simulink library "carnotUIBK"  (R2024b)
settings: Solver=VariableStepAuto  StartTime=0.0  StopTime=10.0  RelTol=1e-3  EnableMultiTasking=on
values from neighbouring files (symbols this model uses):
  area = area + room(kk).area    [THERMALZONE.m]
  boundary = BOUNDARY()    [BUILDING.m]
  building = obj    [BUILDING.m]
  C = zeros(1,length(d)+1)    [CONSTRUCTION.m]
  cp = str2num(value)    [CONSTRUCTION.m]
  pos = find(d_layer>0)    [CONSTRUCTION.m]
  rho = str2num(value)    [CONSTRUCTION.m]
  type = 1    [CONSTRUCTION.m]
  zone = obj.zone(ind)    [THERMALZONE.m]
undefined symbols (not defined in the file or in its folder): A, amb_factor, B, const, control, Dd, get_building, height, p, Qdot_C, Qdot_H, Qdot_I_electricity, Qdot_I_light, Qdot_I_person, Qdot_S, Qdot_T_ground, Qdot_T_neighbour, Qdot_T_opaque, Qdot_T_window, Qdot_V_infiltration, Qdot_V_mech, Qdot_V_window, r_frame, solar_ratio, solar_ratio1, solar_ratio2, Tc, Tr, Ts, Uvalue, view_factor, wall, wallsurface, window, window_height, window_heigth, window_width, windowsurface, x_CO2, x_H2O, x_VOC, z
libraries: carnot x105, $bdroot x22, simulink x18, simulink_extras x14
(part 8 of 13)

== system carnotUIBK/window/window_CARNOT/alfa_window_in ==
  note: (W/m^2)
  note: CONVENTION:
      | Qdot > 0 and qdots < 0, if Ts > T (heat flows from wall surface to room node),
      | Qdot < 0 and qdots > 0, if Ts < T (heat flows from room node to wall surface).
  note: s: surface
      | c: convective
      | r: radiative
  note: WINDOW = FRAME + GLASS
  note: (W/m^2)
  note: Convective and radiative heat transfer at the INDOOR SURFACE OF A VERTICAL WINDOW
      | with 1-4 layers (each 3 ... 8 mm thick)
  note: (°C)
  Ts2 : Inport
  "[sun_t]" : Inport  Port=2
  "[AIV]" : Inport  Port=3
  Demux : Demux  Outputs=[1 1 1 6]
      settings: DisplayOption=none
  Demux1 : Demux  Outputs=[1 2]
      settings: DisplayOption=none
  Ground2 : Ground
  Ground3 : Ground
  Ground4 : Ground
  Irradiation into room : Subsystem
  Mux : Mux  Inputs=2
  Mux4 : Mux  Inputs=[2 1 2 2 12]
  Product5 : Product  InputSameDT=on  SaturateOnIntegerOverflow=on  OutDataTypeStr=Inherit: Same as first input
  Sum : Sum  Inputs=-+  InputSameDT=on  SaturateOnIntegerOverflow=on  OutDataTypeStr=Inherit: Same as first input
  Sum1 : Sum  Inputs=+-  InputSameDT=on  SaturateOnIntegerOverflow=on  OutDataTypeStr=Inherit: Same as first input
  Sum2 : Sum  Inputs=--  InputSameDT=on  SaturateOnIntegerOverflow=on  OutDataTypeStr=Inherit: Same as first input
  Terminator : Terminator
  Terminator1 : Terminator
  emission_in : Gain  Gain=emission_in  SaturateOnIntegerOverflow=on  OutDataTypeStr=Inherit: Same as input  ParamDataTypeStr=Inherit: Same as input
  surface of window : Gain  Gain=wallsurface  SaturateOnIntegerOverflow=on  OutDataTypeStr=Inherit: Same as input  ParamDataTypeStr=Inherit: Same as input
  surface of window glass : Gain  Gain=(1-frame)*wallsurface  SaturateOnIntegerOverflow=on  OutDataTypeStr=Inherit: Same as input  ParamDataTypeStr=Inherit: Same as input
  transmission coefficient 1-2-3-4-layer(s) : Subsystem
  u_convection : Gain  Gain=2.5  SaturateOnIntegerOverflow=on  OutDataTypeStr=Inherit: Same as input  ParamDataTypeStr=Inherit: Same as input
  u_rad : Constant  Value=5.6
  u_rad1 : Constant  Value=zeros(numlayer,1)
  qdots2 : Outport  InitialOutput=0  VectorParamsAs1DForOutWhenUnconnected=off
  qdot_abs : Outport  Port=2  InitialOutput=0  VectorParamsAs1DForOutWhenUnconnected=off
  "[S]" : Outport  Port=3  InitialOutput=0  VectorParamsAs1DForOutWhenUnconnected=off
  wires:
  Sum2/1 -> qdots2/1
  Demux/4 -> Terminator1/1
  "[AIV]"/1 -> Demux/1
  Demux/1 -> Terminator/1
  Mux/1 -> surface of window/1
  emission_in/1 -> Product5/1
  Sum1/1 -> Product5/2  "dTr"
  u_rad/1 -> emission_in/1
  Ts2/1 -> Sum/2, Sum1/1  "Ts"
  Product5/1 -> Mux/2, Sum2/2  "qdotr"
  u_convection/1 -> Sum2/1, Mux/1  "qdotc"
  Irradiation into room/1(qdot_sol) -> surface of window glass/1  "qdot_sol (>= 0)"
  Demux1/1 -> transmission coefficient 1-2-3-4-layer(s)/1(teta)  "teta"
  "[sun_t]"/1 -> Demux1/1
  Demux/2 -> Sum/1  "Tc"
  u_rad1/1 -> qdot_abs/1
  Sum/1 -> u_convection/1  "dTc"
  Demux/3 -> Sum1/2  "Tr"
  Demux1/2 -> Irradiation into room/1("[I_t]")  "[I_t]"
  transmission coefficient 1-2-3-4-layer(s)/1("[tau]") -> Irradiation into room/2("[tau]")
  Mux4/1 -> "[S]"/1
  Ground3/1 -> Mux4/5
  Ground2/1 -> Mux4/4
  Ground4/1 -> Mux4/3
  surface of window/1 -> Mux4/1  "[Qdotc, Qdotr]"
  surface of window glass/1 -> Mux4/2  "Qdot_sol"

== system carnotUIBK/window/window_CARNOT/alfa_window_out ==
  note: WINDOW = FRAME + GLASS
  note: Convective and radiative heat transfer at the OUTDOOR SURFACE OF A VERTICAL WINDOW
  note: modified
      | weatherdata
  note: s: surface
      | c: convective
      | r: radiative
      | h: in height
      | t: tilted surface
  note: CONVENTION:
      | qdots < 0, if Ts > T, heat flows from window surface (resp. room node) to ambition,
      | qdots > 0, if Ts < T, heat flows from ambition to window surface (resp. room node).
  WDB : Inport
  g : Inport  Port=2
  Ts1 : Inport  Port=3
  Bus Selector : BusSelector  OutputSignals=Temperature_Ambient,Temperature_Sky_Radiation,Wind_Speed
  Bus Selector1 : BusSelector  OutputSignals=Incidence_Angle_sun,Solar_Radiation_direct_surface,Solar_Radiation_diffuse_surface
  Ground1 : Ground
  Ground2 : Ground
  Ground3 : Ground
  Mux1 : Mux  Inputs=2
  Mux2 : Mux  Inputs=2
  Mux3 : Mux  Inputs=[1 1 5 3 1 8]
  Product6 : Product  InputSameDT=on  SaturateOnIntegerOverflow=on  OutDataTypeStr=Inherit: Same as first input
  Product7 : Product  InputSameDT=on  SaturateOnIntegerOverflow=on  OutDataTypeStr=Inherit: Same as first input
  Qdotc : Constant  Value=0
  Qdotr : Constant  Value=0
  Radiation_on_Inclined_Surface : carnot/Weather/Radiation_on_Inclined_Surface  sky=Perez 1990  reflect=0.2
      settings: SourceProductName=Carnot
  Sum : Sum  Inputs=+-  InputSameDT=on  SaturateOnIntegerOverflow=on  OutDataTypeStr=Inherit: Same as first input
  Sum2 : Sum  Inputs=+++  InputSameDT=on  SaturateOnIntegerOverflow=on  OutDataTypeStr=Inherit: Same as first input
  Sum3 : Sum  InputSameDT=on  SaturateOnIntegerOverflow=on  OutDataTypeStr=Inherit: Same as first input
  absorption_out * frame : Gain  Gain=absorption_out * frame  SaturateOnIntegerOverflow=on  OutDataTypeStr=Inherit: Same as input  ParamDataTypeStr=Inherit: Same as input
  alfa : Fcn  Expr=3*u(1)+2.8
  position : Constant  Value=pos
  qp rad : Subsystem
  surface of window : Gain  Gain=windowsurface  SaturateOnIntegerOverflow=on  OutDataTypeStr=Inherit: Same as input  ParamDataTypeStr=Inherit: Same as input
  "[sun_t]" : Outport  InitialOutput=0  VectorParamsAs1DForOutWhenUnconnected=off
  qdots1 : Outport  Port=2  InitialOutput=0  VectorParamsAs1DForOutWhenUnconnected=off
  "[S]" : Outport  Port=3  InitialOutput=0  VectorParamsAs1DForOutWhenUnconnected=off
  wires:
  Radiation_on_Inclined_Surface/1 -> Bus Selector1/1
  position/1 -> Radiation_on_Inclined_Surface/2
  Product7/1 -> Sum2/1  "qdot,conv"
  alfa/1 -> Product7/2  "alfa"
  qp rad/1(qprad) -> Sum2/2  "qdotr"
  Ts1/1 -> qp rad/2(Tw), Sum/2  "Ts (outer wall surface)"
  Mux1/1 -> "[sun_t]"/1
  Bus Selector1/2 -> Mux2/1, Sum3/1  "<Solar_Radiation_direct_surface>"
  absorption_out * frame/1 -> Sum2/3
  g/1 -> Product6/2
  Sum2/1 -> surface of window/1, qdots1/1
  Sum3/1 -> absorption_out * frame/1
  Bus Selector1/1 -> Mux1/1  "<Incidence_Angle_sun>"
  WDB/1 -> Radiation_on_Inclined_Surface/1, Bus Selector/1
  Sum/1 -> Product7/1  "dTc"
  Product6/1 -> Mux1/2
  Mux2/1 -> Product6/1
  Bus Selector1/3 -> Mux2/2, Sum3/2  "<Solar_Radiation_diffuse_surface>"
  Bus Selector/1 -> qp rad/1(Ta), Sum/1  "<Temperature_Ambient>"
  Bus Selector/2 -> qp rad/3(Tsky)  "<Temperature_Sky_Radiation>"
  Bus Selector/3 -> alfa/1  "<Wind_Speed>"
  Mux3/1 -> "[S]"/1
  Ground2/1 -> Mux3/6
  Ground3/1 -> Mux3/3
  Qdotc/1 -> Mux3/1
  Qdotr/1 -> Mux3/2
  Ground1/1 -> Mux3/4
  surface of window/1 -> Mux3/5

== system carnotUIBK/window/window_TF/alfa_window_in ==
  note: Convective and radiative heat transfer at the INDOOR SURFACE OF A VERTICAL WINDOW
      | with 1-4 layers (each 3 ... 8 mm thick)
  note: WINDOW = FRAME + GLASS
  note: s: surface
      | c: convective
      | r: radiative
  note: CONVENTION:
      | Qdot > 0 and qdots < 0, if Ts > T (heat flows from wall surface to room node),
      | Qdot < 0 and qdots > 0, if Ts < T (heat flows from room node to wall surface).
  note: (W/m^2)
  Ts2 : Inport
  "[sun_t]" : Inport  Port=2
  "[AIV]" : Inport  Port=3
  WDB : Inport  Port=4
  control : Inport  Port=5
  Bus Selector : BusSelector  OutputSignals=Tc,Tr
  Fcn : Fcn  Expr=1.6*(abs(u(1)-u(2)))^0.3
  Fcn1 : Fcn  Expr=(273.15+u(1))^4-(273.15+u(2))^4
  Ground2 : Ground
  Ground3 : Ground
  Ground4 : Ground
  Mux : Mux  Inputs=2
  Mux2 : Mux  Inputs=2
  Mux3 : Mux  Inputs=2
  Mux4 : Mux  Inputs=[2 1 2 2 12]
  Product : Product  InputSameDT=on  RndMeth=Zero  SaturateOnIntegerOverflow=on  OutDataTypeStr=Inherit: Same as first input
  Product1 : Product  InputSameDT=on  RndMeth=Zero  SaturateOnIntegerOverflow=on  OutDataTypeStr=Inherit: Same as first input
  Sum : Sum  Inputs=+-  InputSameDT=on  SaturateOnIntegerOverflow=on  OutDataTypeStr=Inherit: Same as first input
  Sum2 : Sum  Inputs=--+  InputSameDT=on  SaturateOnIntegerOverflow=on  OutDataTypeStr=Inherit: Same as first input
  emission_in : Gain  Gain=emission_in  SaturateOnIntegerOverflow=on  OutDataTypeStr=Inherit: Same as input  ParamDataTypeStr=Inherit: Same as input
  glass ratio : Gain  Gain=(1-frame)  SaturateOnIntegerOverflow=on  OutDataTypeStr=Inherit: Same as input  ParamDataTypeStr=Inherit: Same as input
  sigma : Constant  Value=5.67e-8
  surface of window : Gain  Gain=windowsurface  SaturateOnIntegerOverflow=on  OutDataTypeStr=Inherit: Same as input  ParamDataTypeStr=Inherit: Same as input
  surface of window glass : Gain  Gain=(1-frame)*windowsurface  SaturateOnIntegerOverflow=on  OutDataTypeStr=Inherit: Same as input  ParamDataTypeStr=Inherit: Same as input
  transmission_absorption : Subsystem
  view_factor : Gain  Gain=view_factor  SaturateOnIntegerOverflow=on  OutDataTypeStr=Inherit: Same as input  ParamDataTypeStr=Inherit: Same as input
  qdots2 : Outport  VectorParamsAs1DForOutWhenUnconnected=off
  "[S]" : Outport  Port=2  VectorParamsAs1DForOutWhenUnconnected=off
  wires:
  control/1 -> transmission_absorption/3(control)
  WDB/1 -> transmission_absorption/2(WDB)
  transmission_absorption/1(qdot_abs) -> glass ratio/1  "qabs"
  transmission_absorption/2(qdot_sol) -> surface of window glass/1  "qdot_sol (>=0)"
  surface of window/1 -> Mux4/1  "[Qdotc, Qdotr]"
  surface of window glass/1 -> Mux4/2  "Qdot_sol"
  "[sun_t]"/1 -> transmission_absorption/1(sun_t)
  Product/1 -> Sum2/2, Mux/2  "qdotr"
  Mux/1 -> surface of window/1
  Sum2/1 -> qdots2/1
  emission_in/1 -> view_factor/1
  sigma/1 -> emission_in/1
  Fcn1/1 -> Product/2
  view_factor/1 -> Product/1
  "[AIV]"/1 -> Bus Selector/1
  Mux3/1 -> Fcn1/1
  Bus Selector/2 -> Mux3/2  "<Tr>"
  Fcn/1 -> Product1/2  "hc"
  Mux2/1 -> Fcn/1
  Sum/1 -> Product1/1  "dTc"
  Ts2/1 -> Sum/1, Mux2/1, Mux3/1  "Ts"
  Bus Selector/1 -> Sum/2, Mux2/2  "<Tc>"
  Product1/1 -> Mux/1, Sum2/1  "qdotc"
  Mux4/1 -> "[S]"/1
  Ground3/1 -> Mux4/5
  Ground2/1 -> Mux4/4
  Ground4/1 -> Mux4/3
  glass ratio/1 -> Sum2/3  "Qdot_sol"

== system carnotUIBK/window/window_TF/alfa_window_out ==
  note: WINDOW = FRAME + GLASS
  note: Convective and radiative heat transfer at the OUTDOOR SURFACE OF A VERTICAL WINDOW
  note: modified
      | weatherdata
  note: s: surface
      | c: convective
      | r: radiative
      | h: in height
      | t: tilted surface
  note: CONVENTION:
      | qdots < 0, if Ts > T, heat flows from window surface (resp. room node) to ambition,
      | qdots > 0, if Ts < T, heat flows from ambition to window surface (resp. room node).
  WDB : Inport
  g : Inport  Port=2
  Ts1 : Inport  Port=3
  Bus Selector : BusSelector  OutputSignals=Temperature_Ambient,Temperature_Sky_Radiation,Wind_Speed
  Bus Selector1 : BusSelector  OutputSignals=Incidence_Angle_sun,Solar_Radiation_direct_surface,Solar_Radiation_diffuse_surface
  Ground1 : Ground
  Ground2 : Ground
  Ground3 : Ground
  Mux1 : Mux  Inputs=2
  Mux2 : Mux  Inputs=2
  Mux3 : Mux  Inputs=[1 1 5 3 1 8]
  Product6 : Product  InputSameDT=on  SaturateOnIntegerOverflow=on  OutDataTypeStr=Inherit: Same as first input
  Product7 : Product  InputSameDT=on  SaturateOnIntegerOverflow=on  OutDataTypeStr=Inherit: Same as first input
  Qdotc : Constant  Value=0
  Qdotr : Constant  Value=0
  Radiation_on_Inclined_Surface : carnot/Weather/Radiation_on_Inclined_Surface  sky=Perez 1990  reflect=0.2
      settings: SourceProductName=Carnot
  Sum : Sum  Inputs=+-  InputSameDT=on  SaturateOnIntegerOverflow=on  OutDataTypeStr=Inherit: Same as first input
  Sum2 : Sum  Inputs=+++  InputSameDT=on  SaturateOnIntegerOverflow=on  OutDataTypeStr=Inherit: Same as first input
  Sum3 : Sum  InputSameDT=on  SaturateOnIntegerOverflow=on  OutDataTypeStr=Inherit: Same as first input
  absorption_out * frame : Gain  Gain=absorption_out * frame  SaturateOnIntegerOverflow=on  OutDataTypeStr=Inherit: Same as input  ParamDataTypeStr=Inherit: Same as input
  alfa : Fcn  Expr=3*u(1)+2.8
  position : Constant  Value=pos
  qp rad : Subsystem
  surface of window : Gain  Gain=windowsurface  SaturateOnIntegerOverflow=on  OutDataTypeStr=Inherit: Same as input  ParamDataTypeStr=Inherit: Same as input
  "[sun_t]" : Outport  InitialOutput=0  VectorParamsAs1DForOutWhenUnconnected=off
  qdots1 : Outport  Port=2  InitialOutput=0  VectorParamsAs1DForOutWhenUnconnected=off
  "[S]" : Outport  Port=3  InitialOutput=0  VectorParamsAs1DForOutWhenUnconnected=off
  wires:
  Radiation_on_Inclined_Surface/1 -> Bus Selector1/1
  position/1 -> Radiation_on_Inclined_Surface/2
  Product7/1 -> Sum2/1  "qdot,conv"
  alfa/1 -> Product7/2  "alfa"
  qp rad/1(qprad) -> Sum2/2  "qdotr"
  Ts1/1 -> qp rad/2(Tw), Sum/2  "Ts (outer wall surface)"
  Mux1/1 -> "[sun_t]"/1
  Bus Selector1/2 -> Mux2/1, Sum3/1  "<Solar_Radiation_direct_surface>"
  absorption_out * frame/1 -> Sum2/3
  g/1 -> Product6/2
  Sum2/1 -> surface of window/1, qdots1/1
  Sum3/1 -> absorption_out * frame/1
  Bus Selector1/1 -> Mux1/1  "<Incidence_Angle_sun>"
  WDB/1 -> Radiation_on_Inclined_Surface/1, Bus Selector/1
  Sum/1 -> Product7/1  "dTc"
  Product6/1 -> Mux1/2
  Mux2/1 -> Product6/1
  Bus Selector1/3 -> Mux2/2, Sum3/2  "<Solar_Radiation_diffuse_surface>"
  Bus Selector/1 -> qp rad/1(Ta), Sum/1  "<Temperature_Ambient>"
  Bus Selector/2 -> qp rad/3(Tsky)  "<Temperature_Sky_Radiation>"
  Bus Selector/3 -> alfa/1  "<Wind_Speed>"
  Mux3/1 -> "[S]"/1
  Ground2/1 -> Mux3/6
  Ground3/1 -> Mux3/3
  Qdotc/1 -> Mux3/1
  Qdotr/1 -> Mux3/2
  Ground1/1 -> Mux3/4
  surface of window/1 -> Mux3/5

== system carnotUIBK/window/window_TF/lambda_window ==
  note: Heat conduction in a window (ONLY SURFACE LAYER CONNECTABLE)
  note: Timeconstant of window is calculated
      | in the mask initialization
  qdots1 : Inport
  qdots2 : Inport  Port=2
  Product1 : Product  InputSameDT=on  RndMeth=Zero  SaturateOnIntegerOverflow=on  OutDataTypeStr=Inherit: Same as first input
  Product6 : Product  InputSameDT=on  RndMeth=Zero  SaturateOnIntegerOverflow=on  OutDataTypeStr=Inherit: Same as first input
  R_win : Constant  Value=Rwin
  Sum1 : Sum  InputSameDT=on  SaturateOnIntegerOverflow=on  OutDataTypeStr=Inherit: Same as first input
  Sum3 : Sum  InputSameDT=on  SaturateOnIntegerOverflow=on  OutDataTypeStr=Inherit: Same as first input
  Transfer Fcn : TransferFcn  Denominator=[timeconst 1]
  Transfer Fcn1 : TransferFcn  Denominator=[timeconst 1]
  Ts1 : Outport  VectorParamsAs1DForOutWhenUnconnected=off
  Ts2 : Outport  Port=2  VectorParamsAs1DForOutWhenUnconnected=off
  wires:
  Transfer Fcn1/1 -> Ts2/1, Sum3/2
  Transfer Fcn/1 -> Ts1/1, Sum1/2
  qdots1/1 -> Product6/2
  qdots2/1 -> Product1/2
  Product6/1 -> Sum3/1
  Sum3/1 -> Transfer Fcn/1
  Product1/1 -> Sum1/1
  Sum1/1 -> Transfer Fcn1/1
  R_win/1 -> Product6/1, Product1/1  "R_win"

== system carnotUIBK/window/window_TF_shading/alfa_window_in ==
  note: Convective and radiative heat transfer at the INDOOR SURFACE OF A VERTICAL WINDOW
      | with 1-4 layers (each 3 ... 8 mm thick)
  note: WINDOW = FRAME + GLASS
  note: s: surface
      | c: convective
      | r: radiative
  note: CONVENTION:
      | Qdot > 0 and qdots < 0, if Ts > T (heat flows from wall surface to room node),
      | Qdot < 0 and qdots > 0, if Ts < T (heat flows from room node to wall surface).
  note: (W/m^2)
  Ts2 : Inport
  "[sun_t]" : Inport  Port=2
  "[AIV]" : Inport  Port=3
  WDB : Inport  Port=4
  control : Inport  Port=5
  Bus Selector : BusSelector  OutputSignals=Tc,Tr
  Fcn : Fcn  Expr=1.6*(abs(u(1)-u(2)))^0.3
  Fcn1 : Fcn  Expr=(273.15+u(1))^4-(273.15+u(2))^4
  Ground2 : Ground
  Ground3 : Ground
  Ground4 : Ground
  Mux : Mux  Inputs=2
  Mux2 : Mux  Inputs=2
  Mux3 : Mux  Inputs=2
  Mux4 : Mux  Inputs=[2 1 2 2 12]
  Product : Product  InputSameDT=on  RndMeth=Zero  SaturateOnIntegerOverflow=on  OutDataTypeStr=Inherit: Same as first input
  Product1 : Product  InputSameDT=on  RndMeth=Zero  SaturateOnIntegerOverflow=on  OutDataTypeStr=Inherit: Same as first input
  Sum : Sum  Inputs=+-  InputSameDT=on  SaturateOnIntegerOverflow=on  OutDataTypeStr=Inherit: Same as first input
  Sum2 : Sum  Inputs=--+  InputSameDT=on  SaturateOnIntegerOverflow=on  OutDataTypeStr=Inherit: Same as first input
  emission_in : Gain  Gain=emission_in  SaturateOnIntegerOverflow=on  OutDataTypeStr=Inherit: Same as input  ParamDataTypeStr=Inherit: Same as input
  sigma : Constant  Value=5.67e-8
  surface of window : Gain  Gain=windowsurface  SaturateOnIntegerOverflow=on  OutDataTypeStr=Inherit: Same as input  ParamDataTypeStr=Inherit: Same as input
  surface of window glass : Gain  Gain=(1-frame)*windowsurface  SaturateOnIntegerOverflow=on  OutDataTypeStr=Inherit: Same as input  ParamDataTypeStr=Inherit: Same as input
  transmission_absorption : Subsystem
  view_factor : Gain  Gain=view_factor  SaturateOnIntegerOverflow=on  OutDataTypeStr=Inherit: Same as input  ParamDataTypeStr=Inherit: Same as input
  qdots2 : Outport  VectorParamsAs1DForOutWhenUnconnected=off
  "[S]" : Outport  Port=2  VectorParamsAs1DForOutWhenUnconnected=off
  wires:
  control/1 -> transmission_absorption/3(control)
  WDB/1 -> transmission_absorption/2(WDB)
  transmission_absorption/1(qdot_abs) -> Sum2/3  "qabs"
  transmission_absorption/2(qdot_sol) -> surface of window glass/1  "qdot_sol (>=0)"
  surface of window/1 -> Mux4/1  "[Qdotc, Qdotr]"
  surface of window glass/1 -> Mux4/2  "Qdot_sol"
  "[sun_t]"/1 -> transmission_absorption/1(sun_t)
  Product/1 -> Sum2/2, Mux/2  "qdotr"
  Mux/1 -> surface of window/1
  Sum2/1 -> qdots2/1
  emission_in/1 -> view_factor/1
  sigma/1 -> emission_in/1
  Fcn1/1 -> Product/2
  view_factor/1 -> Product/1
  "[AIV]"/1 -> Bus Selector/1
  Mux3/1 -> Fcn1/1
  Bus Selector/2 -> Mux3/2  "<Tr>"
  Fcn/1 -> Product1/2  "hc"
  Mux2/1 -> Fcn/1
  Sum/1 -> Product1/1  "dTc"
  Ts2/1 -> Sum/1, Mux2/1, Mux3/1  "Ts"
  Bus Selector/1 -> Sum/2, Mux2/2  "<Tc>"
  Product1/1 -> Mux/1, Sum2/1  "qdotc"
  Mux4/1 -> "[S]"/1
  Ground3/1 -> Mux4/5
  Ground2/1 -> Mux4/4
  Ground4/1 -> Mux4/3

== system carnotUIBK/window/window_TF_shading/alfa_window_out ==
  note: WINDOW = FRAME + GLASS
  note: Convective and radiative heat transfer at the OUTDOOR SURFACE OF A VERTICAL WINDOW
  note: modified
      | weatherdata
  note: s: surface
      | c: convective
      | r: radiative
      | h: in height
      | t: tilted surface
  note: CONVENTION:
      | qdots < 0, if Ts > T, heat flows from window surface (resp. room node) to ambition,
      | qdots > 0, if Ts < T, heat flows from ambition to window surface (resp. room node).
  WDB : Inport
  g : Inport  Port=2
  Ts1 : Inport  Port=3
  Bus Selector : BusSelector  OutputSignals=Temperature_Ambient,Temperature_Sky_Radiation,Wind_Speed
  Bus Selector1 : BusSelector  OutputSignals=Incidence_Angle_sun,Solar_Radiation_direct_surface,Solar_Radiation_diffuse_surface
  Ground1 : Ground
  Ground2 : Ground
  Ground3 : Ground
  Mux1 : Mux  Inputs=2
  Mux2 : Mux  Inputs=2
  Mux3 : Mux  Inputs=[1 1 5 3 1 8]
  Product6 : Product  InputSameDT=on  SaturateOnIntegerOverflow=on  OutDataTypeStr=Inherit: Same as first input
  Product7 : Product  InputSameDT=on  SaturateOnIntegerOverflow=on  OutDataTypeStr=Inherit: Same as first input
  Qdotc : Constant  Value=0
  Qdotr : Constant  Value=0
  Radiation_on_Inclined_Surface : carnot/Weather/Radiation_on_Inclined_Surface  sky=Perez 1990  reflect=0.2
      settings: SourceProductName=Carnot
  Sum : Sum  Inputs=+-  InputSameDT=on  SaturateOnIntegerOverflow=on  OutDataTypeStr=Inherit: Same as first input
  Sum2 : Sum  Inputs=+++  InputSameDT=on  SaturateOnIntegerOverflow=on  OutDataTypeStr=Inherit: Same as first input
  Sum3 : Sum  InputSameDT=on  SaturateOnIntegerOverflow=on  OutDataTypeStr=Inherit: Same as first input
  absorption_out * frame : Gain  Gain=absorption_out * frame  SaturateOnIntegerOverflow=on  OutDataTypeStr=Inherit: Same as input  ParamDataTypeStr=Inherit: Same as input
  alfa : Fcn  Expr=3*u(1)+2.8
  position : Constant  Value=pos
  qp rad : Subsystem
  surface of window : Gain  Gain=windowsurface  SaturateOnIntegerOverflow=on  OutDataTypeStr=Inherit: Same as input  ParamDataTypeStr=Inherit: Same as input
  "[sun_t]" : Outport  InitialOutput=0  VectorParamsAs1DForOutWhenUnconnected=off
  qdots1 : Outport  Port=2  InitialOutput=0  VectorParamsAs1DForOutWhenUnconnected=off
  "[S]" : Outport  Port=3  InitialOutput=0  VectorParamsAs1DForOutWhenUnconnected=off
  wires:
  Radiation_on_Inclined_Surface/1 -> Bus Selector1/1
  position/1 -> Radiation_on_Inclined_Surface/2
  Product7/1 -> Sum2/1  "qdot,conv"
  alfa/1 -> Product7/2  "alfa"
  qp rad/1(qprad) -> Sum2/2  "qdotr"
  Ts1/1 -> qp rad/2(Tw), Sum/2  "Ts (outer wall surface)"
  Mux1/1 -> "[sun_t]"/1
  Bus Selector1/2 -> Mux2/1, Sum3/1  "<Solar_Radiation_direct_surface>"
  absorption_out * frame/1 -> Sum2/3
  g/1 -> Product6/2
  Sum2/1 -> surface of window/1, qdots1/1
  Sum3/1 -> absorption_out * frame/1
  Bus Selector1/1 -> Mux1/1  "<Incidence_Angle_sun>"
  WDB/1 -> Radiation_on_Inclined_Surface/1, Bus Selector/1
  Sum/1 -> Product7/1  "dTc"
  Product6/1 -> Mux1/2
  Mux2/1 -> Product6/1
  Bus Selector1/3 -> Mux2/2, Sum3/2  "<Solar_Radiation_diffuse_surface>"
  Bus Selector/1 -> qp rad/1(Ta), Sum/1  "<Temperature_Ambient>"
  Bus Selector/2 -> qp rad/3(Tsky)  "<Temperature_Sky_Radiation>"
  Bus Selector/3 -> alfa/1  "<Wind_Speed>"
  Mux3/1 -> "[S]"/1
  Ground2/1 -> Mux3/6
  Ground3/1 -> Mux3/3
  Qdotc/1 -> Mux3/1
  Qdotr/1 -> Mux3/2
  Ground1/1 -> Mux3/4
  surface of window/1 -> Mux3/5

== system carnotUIBK/window/window_TF_shading/lambda_window ==
  note: Heat conduction in a window (ONLY SURFACE LAYER CONNECTABLE)
  note: Timeconstant of window is calculated
      | in the mask initialization
  qdots1 : Inport
  qdots2 : Inport  Port=2
  Product1 : Product  InputSameDT=on  RndMeth=Zero  SaturateOnIntegerOverflow=on  OutDataTypeStr=Inherit: Same as first input
  Product6 : Product  InputSameDT=on  RndMeth=Zero  SaturateOnIntegerOverflow=on  OutDataTypeStr=Inherit: Same as first input
  R_win : Constant  Value=Rwin
  Sum1 : Sum  InputSameDT=on  SaturateOnIntegerOverflow=on  OutDataTypeStr=Inherit: Same as first input
  Sum3 : Sum  InputSameDT=on  SaturateOnIntegerOverflow=on  OutDataTypeStr=Inherit: Same as first input
  Transfer Fcn : TransferFcn  Denominator=[timeconst 1]
  Transfer Fcn1 : TransferFcn  Denominator=[timeconst 1]
  Ts1 : Outport  VectorParamsAs1DForOutWhenUnconnected=off
  Ts2 : Outport  Port=2  VectorParamsAs1DForOutWhenUnconnected=off
  wires:
  Transfer Fcn1/1 -> Ts2/1, Sum3/2
  Transfer Fcn/1 -> Ts1/1, Sum1/2
  qdots1/1 -> Product6/2
  qdots2/1 -> Product1/2
  Product6/1 -> Sum3/1
  Sum3/1 -> Transfer Fcn/1
  Product1/1 -> Sum1/1
  Sum1/1 -> Transfer Fcn1/1
  R_win/1 -> Product6/1, Product1/1  "R_win"

== system carnotUIBK/HVAC/HVAC_1001_electrical heaters/electrical heater zone 1/Transfer Fcn (with initial states) ==
  In1 : Inport
  State Space : StateSpace  A=A  B=B  C=C  D=Dd  InitialCondition=X0
  Out1 : Outport  InitialOutput=0  VectorParamsAs1DForOutWhenUnconnected=off
  wires:
  In1/1 -> State Space/1
  State Space/1 -> Out1/1

== system carnotUIBK/HVAC/HVAC_1001_electrical heaters/electrical heater zone 10/Transfer Fcn (with initial states) ==
  In1 : Inport
  State Space : StateSpace  A=A  B=B  C=C  D=Dd  InitialCondition=X0
  Out1 : Outport  InitialOutput=0  VectorParamsAs1DForOutWhenUnconnected=off
  wires:
  State Space/1 -> Out1/1
  In1/1 -> State Space/1

== system carnotUIBK/HVAC/HVAC_1001_electrical heaters/electrical heater zone 2/Transfer Fcn (with initial states) ==
  In1 : Inport
  State Space : StateSpace  A=A  B=B  C=C  D=Dd  InitialCondition=X0
  Out1 : Outport  InitialOutput=0  VectorParamsAs1DForOutWhenUnconnected=off
  wires:
  State Space/1 -> Out1/1
  In1/1 -> State Space/1

== system carnotUIBK/HVAC/HVAC_1001_electrical heaters/electrical heater zone 3/Transfer Fcn (with initial states) ==
  In1 : Inport
  State Space : StateSpace  A=A  B=B  C=C  D=Dd  InitialCondition=X0
  Out1 : Outport  InitialOutput=0  VectorParamsAs1DForOutWhenUnconnected=off
  wires:
  In1/1 -> State Space/1
  State Space/1 -> Out1/1

== system carnotUIBK/HVAC/HVAC_1001_electrical heaters/electrical heater zone 4/Transfer Fcn (with initial states) ==
  In1 : Inport
  State Space : StateSpace  A=A  B=B  C=C  D=Dd  InitialCondition=X0
  Out1 : Outport  InitialOutput=0  VectorParamsAs1DForOutWhenUnconnected=off
  wires:
  State Space/1 -> Out1/1
  In1/1 -> State Space/1

== system carnotUIBK/HVAC/HVAC_1001_electrical heaters/electrical heater zone 5/Transfer Fcn (with initial states) ==
  In1 : Inport
  State Space : StateSpace  A=A  B=B  C=C  D=Dd  InitialCondition=X0
  Out1 : Outport  InitialOutput=0  VectorParamsAs1DForOutWhenUnconnected=off
  wires:
  In1/1 -> State Space/1
  State Space/1 -> Out1/1

== system carnotUIBK/HVAC/HVAC_1001_electrical heaters/electrical heater zone 6/Transfer Fcn (with initial states) ==
  In1 : Inport
  State Space : StateSpace  A=A  B=B  C=C  D=Dd  InitialCondition=X0
  Out1 : Outport  InitialOutput=0  VectorParamsAs1DForOutWhenUnconnected=off
  wires:
  State Space/1 -> Out1/1
  In1/1 -> State Space/1

== system carnotUIBK/HVAC/HVAC_1001_electrical heaters/electrical heater zone 7/Transfer Fcn (with initial states) ==
  In1 : Inport
  State Space : StateSpace  A=A  B=B  C=C  D=Dd  InitialCondition=X0
  Out1 : Outport  InitialOutput=0  VectorParamsAs1DForOutWhenUnconnected=off
  wires:
  In1/1 -> State Space/1
  State Space/1 -> Out1/1

== system carnotUIBK/HVAC/HVAC_1001_electrical heaters/electrical heater zone 8/Transfer Fcn (with initial states) ==
  In1 : Inport
  State Space : StateSpace  A=A  B=B  C=C  D=Dd  InitialCondition=X0
  Out1 : Outport  InitialOutput=0  VectorParamsAs1DForOutWhenUnconnected=off
  wires:
  State Space/1 -> Out1/1
  In1/1 -> State Space/1

== system carnotUIBK/HVAC/HVAC_1001_electrical heaters/electrical heater zone 9/Transfer Fcn (with initial states) ==
  In1 : Inport
  State Space : StateSpace  A=A  B=B  C=C  D=Dd  InitialCondition=X0
  Out1 : Outport  InitialOutput=0  VectorParamsAs1DForOutWhenUnconnected=off
  wires:
  In1/1 -> State Space/1
  State Space/1 -> Out1/1

== system carnotUIBK/HVAC/HVAC_2001_ventilation system simple/ventilation_zone 1/Subsystem ==
  note: (kg/s)
  note: (kg/s)
  note: (kg/s)
  note: (kg/kg)
  note: (kg/kg)
  note: ASSUMPTION: mdot_air_out2in = mdot_air_in2out !
  mdot_air : Inport
  x_in : Inport  Port=2
  x_out : Inport  Port=3
  Demux2 : Demux  Outputs=2
      settings: DisplayOption=none
  Demux3 : Demux  Outputs=2
      settings: DisplayOption=none
  Fcn{,1..3} (4 alike) : Fcn  Expr=u / (1+u)
  Product5 : Product  InputSameDT=on  SaturateOnIntegerOverflow=on  OutDataTypeStr=Inherit: Same as first input
  Product6 : Product  InputSameDT=on  SaturateOnIntegerOverflow=on  OutDataTypeStr=Inherit: Same as first input
  Sum1 : Sum  Inputs=+-  InputSameDT=on  SaturateOnIntegerOverflow=on  OutDataTypeStr=Inherit: Same as first input
  Sum2 : Sum  Inputs=+-  InputSameDT=on  SaturateOnIntegerOverflow=on  OutDataTypeStr=Inherit: Same as first input
  mdot_H2O : Outport  VectorParamsAs1DForOutWhenUnconnected=off
  mdot_CO2 : Outport  Port=2  VectorParamsAs1DForOutWhenUnconnected=off
  wires:
  x_out/1 -> Demux2/1
  Demux2/1 -> Fcn/1  "x_H2O_out"
  Demux2/2 -> Fcn1/1  "x_CO2_out"
  Demux3/2 -> Fcn3/1  "x_CO2_in"
  Demux3/1 -> Fcn2/1  "x_H2O_in"
  x_in/1 -> Demux3/1
  Fcn/1 -> Sum1/1
  Fcn2/1 -> Sum1/2
  Fcn1/1 -> Sum2/1
  Fcn3/1 -> Sum2/2
  Sum2/1 -> Product6/2
  Sum1/1 -> Product5/2
  mdot_air/1 -> Product6/1, Product5/1  "mdot_air >=0"
  Product6/1 -> mdot_CO2/1
  Product5/1 -> mdot_H2O/1

== system carnotUIBK/HVAC/HVAC_2001_ventilation system simple/ventilation_zone 10/Subsystem ==
  note: (kg/s)
  note: (kg/s)
  note: (kg/s)
  note: (kg/kg)
  note: (kg/kg)
  note: ASSUMPTION: mdot_air_out2in = mdot_air_in2out !
  mdot_air : Inport
  x_in : Inport  Port=2
  x_out : Inport  Port=3
  Demux2 : Demux  Outputs=2
      settings: DisplayOption=none
  Demux3 : Demux  Outputs=2
      settings: DisplayOption=none
  Fcn{,1..3} (4 alike) : Fcn  Expr=u / (1+u)
  Product5 : Product  InputSameDT=on  SaturateOnIntegerOverflow=on  OutDataTypeStr=Inherit: Same as first input
  Product6 : Product  InputSameDT=on  SaturateOnIntegerOverflow=on  OutDataTypeStr=Inherit: Same as first input
  Sum1 : Sum  Inputs=+-  InputSameDT=on  SaturateOnIntegerOverflow=on  OutDataTypeStr=Inherit: Same as first input
  Sum2 : Sum  Inputs=+-  InputSameDT=on  SaturateOnIntegerOverflow=on  OutDataTypeStr=Inherit: Same as first input
  mdot_H2O : Outport  VectorParamsAs1DForOutWhenUnconnected=off
  mdot_CO2 : Outport  Port=2  VectorParamsAs1DForOutWhenUnconnected=off
  wires:
  x_out/1 -> Demux2/1
  Demux2/1 -> Fcn/1  "x_H2O_out"
  Demux2/2 -> Fcn1/1  "x_CO2_out"
  Demux3/2 -> Fcn3/1  "x_CO2_in"
  Demux3/1 -> Fcn2/1  "x_H2O_in"
  x_in/1 -> Demux3/1
  Fcn/1 -> Sum1/1
  Fcn2/1 -> Sum1/2
  Fcn1/1 -> Sum2/1
  Fcn3/1 -> Sum2/2
  Sum2/1 -> Product6/2
  Sum1/1 -> Product5/2
  mdot_air/1 -> Product6/1, Product5/1  "mdot_air >=0"
  Product6/1 -> mdot_CO2/1
  Product5/1 -> mdot_H2O/1

== system carnotUIBK/HVAC/HVAC_2001_ventilation system simple/ventilation_zone 2/Subsystem ==
  note: ASSUMPTION: mdot_air_out2in = mdot_air_in2out !
  note: (kg/kg)
  note: (kg/kg)
  note: (kg/s)
  note: (kg/s)
  note: (kg/s)
  mdot_air : Inport
  x_in : Inport  Port=2
  x_out : Inport  Port=3
  Demux2 : Demux  Outputs=2
      settings: DisplayOption=none
  Demux3 : Demux  Outputs=2
      settings: DisplayOption=none
  Fcn{,1..3} (4 alike) : Fcn  Expr=u / (1+u)
  Product5 : Product  InputSameDT=on  SaturateOnIntegerOverflow=on  OutDataTypeStr=Inherit: Same as first input
  Product6 : Product  InputSameDT=on  SaturateOnIntegerOverflow=on  OutDataTypeStr=Inherit: Same as first input
  Sum1 : Sum  Inputs=+-  InputSameDT=on  SaturateOnIntegerOverflow=on  OutDataTypeStr=Inherit: Same as first input
  Sum2 : Sum  Inputs=+-  InputSameDT=on  SaturateOnIntegerOverflow=on  OutDataTypeStr=Inherit: Same as first input
  mdot_H2O : Outport  VectorParamsAs1DForOutWhenUnconnected=off
  mdot_CO2 : Outport  Port=2  VectorParamsAs1DForOutWhenUnconnected=off
  wires:
  Product5/1 -> mdot_H2O/1
  Product6/1 -> mdot_CO2/1
  mdot_air/1 -> Product5/1, Product6/1  "mdot_air >=0"
  Sum1/1 -> Product5/2
  Sum2/1 -> Product6/2
  Fcn3/1 -> Sum2/2
  Fcn1/1 -> Sum2/1
  Fcn2/1 -> Sum1/2
  Fcn/1 -> Sum1/1
  x_in/1 -> Demux3/1
  Demux3/1 -> Fcn2/1  "x_H2O_in"
  Demux3/2 -> Fcn3/1  "x_CO2_in"
  Demux2/2 -> Fcn1/1  "x_CO2_out"
  Demux2/1 -> Fcn/1  "x_H2O_out"
  x_out/1 -> Demux2/1

== system carnotUIBK/HVAC/HVAC_2001_ventilation system simple/ventilation_zone 3/Subsystem ==
  note: (kg/s)
  note: (kg/s)
  note: (kg/s)
  note: (kg/kg)
  note: (kg/kg)
  note: ASSUMPTION: mdot_air_out2in = mdot_air_in2out !
  mdot_air : Inport
  x_in : Inport  Port=2
  x_out : Inport  Port=3
  Demux2 : Demux  Outputs=2
      settings: DisplayOption=none
  Demux3 : Demux  Outputs=2
      settings: DisplayOption=none
  Fcn{,1..3} (4 alike) : Fcn  Expr=u / (1+u)
  Product5 : Product  InputSameDT=on  SaturateOnIntegerOverflow=on  OutDataTypeStr=Inherit: Same as first input
  Product6 : Product  InputSameDT=on  SaturateOnIntegerOverflow=on  OutDataTypeStr=Inherit: Same as first input
  Sum1 : Sum  Inputs=+-  InputSameDT=on  SaturateOnIntegerOverflow=on  OutDataTypeStr=Inherit: Same as first input
  Sum2 : Sum  Inputs=+-  InputSameDT=on  SaturateOnIntegerOverflow=on  OutDataTypeStr=Inherit: Same as first input
  mdot_H2O : Outport  VectorParamsAs1DForOutWhenUnconnected=off
  mdot_CO2 : Outport  Port=2  VectorParamsAs1DForOutWhenUnconnected=off
  wires:
  x_out/1 -> Demux2/1
  Demux2/1 -> Fcn/1  "x_H2O_out"
  Demux2/2 -> Fcn1/1  "x_CO2_out"
  Demux3/2 -> Fcn3/1  "x_CO2_in"
  Demux3/1 -> Fcn2/1  "x_H2O_in"
  x_in/1 -> Demux3/1
  Fcn/1 -> Sum1/1
  Fcn2/1 -> Sum1/2
  Fcn1/1 -> Sum2/1
  Fcn3/1 -> Sum2/2
  Sum2/1 -> Product6/2
  Sum1/1 -> Product5/2
  mdot_air/1 -> Product6/1, Product5/1  "mdot_air >=0"
  Product6/1 -> mdot_CO2/1
  Product5/1 -> mdot_H2O/1

== system carnotUIBK/HVAC/HVAC_2001_ventilation system simple/ventilation_zone 4/Subsystem ==
  note: (kg/s)
  note: (kg/s)
  note: (kg/s)
  note: (kg/kg)
  note: (kg/kg)
  note: ASSUMPTION: mdot_air_out2in = mdot_air_in2out !
  mdot_air : Inport
  x_in : Inport  Port=2
  x_out : Inport  Port=3
  Demux2 : Demux  Outputs=2
      settings: DisplayOption=none
  Demux3 : Demux  Outputs=2
      settings: DisplayOption=none
  Fcn{,1..3} (4 alike) : Fcn  Expr=u / (1+u)
  Product5 : Product  InputSameDT=on  SaturateOnIntegerOverflow=on  OutDataTypeStr=Inherit: Same as first input
  Product6 : Product  InputSameDT=on  SaturateOnIntegerOverflow=on  OutDataTypeStr=Inherit: Same as first input
  Sum1 : Sum  Inputs=+-  InputSameDT=on  SaturateOnIntegerOverflow=on  OutDataTypeStr=Inherit: Same as first input
  Sum2 : Sum  Inputs=+-  InputSameDT=on  SaturateOnIntegerOverflow=on  OutDataTypeStr=Inherit: Same as first input
  mdot_H2O : Outport  VectorParamsAs1DForOutWhenUnconnected=off
  mdot_CO2 : Outport  Port=2  VectorParamsAs1DForOutWhenUnconnected=off
  wires:
  x_out/1 -> Demux2/1
  Demux2/1 -> Fcn/1  "x_H2O_out"
  Demux2/2 -> Fcn1/1  "x_CO2_out"
  Demux3/2 -> Fcn3/1  "x_CO2_in"
  Demux3/1 -> Fcn2/1  "x_H2O_in"
  x_in/1 -> Demux3/1
  Fcn/1 -> Sum1/1
  Fcn2/1 -> Sum1/2
  Fcn1/1 -> Sum2/1
  Fcn3/1 -> Sum2/2
  Sum2/1 -> Product6/2
  Sum1/1 -> Product5/2
  mdot_air/1 -> Product6/1, Product5/1  "mdot_air >=0"
  Product6/1 -> mdot_CO2/1
  Product5/1 -> mdot_H2O/1

== system carnotUIBK/HVAC/HVAC_2001_ventilation system simple/ventilation_zone 5/Subsystem ==
  note: (kg/s)
  note: (kg/s)
  note: (kg/s)
  note: (kg/kg)
  note: (kg/kg)
  note: ASSUMPTION: mdot_air_out2in = mdot_air_in2out !
  mdot_air : Inport
  x_in : Inport  Port=2
  x_out : Inport  Port=3
  Demux2 : Demux  Outputs=2
      settings: DisplayOption=none
  Demux3 : Demux  Outputs=2
      settings: DisplayOption=none
  Fcn{,1..3} (4 alike) : Fcn  Expr=u / (1+u)
  Product5 : Product  InputSameDT=on  SaturateOnIntegerOverflow=on  OutDataTypeStr=Inherit: Same as first input
  Product6 : Product  InputSameDT=on  SaturateOnIntegerOverflow=on  OutDataTypeStr=Inherit: Same as first input
  Sum1 : Sum  Inputs=+-  InputSameDT=on  SaturateOnIntegerOverflow=on  OutDataTypeStr=Inherit: Same as first input
  Sum2 : Sum  Inputs=+-  InputSameDT=on  SaturateOnIntegerOverflow=on  OutDataTypeStr=Inherit: Same as first input
  mdot_H2O : Outport  VectorParamsAs1DForOutWhenUnconnected=off
  mdot_CO2 : Outport  Port=2  VectorParamsAs1DForOutWhenUnconnected=off
  wires:
  x_out/1 -> Demux2/1
  Demux2/1 -> Fcn/1  "x_H2O_out"
  Demux2/2 -> Fcn1/1  "x_CO2_out"
  Demux3/2 -> Fcn3/1  "x_CO2_in"
  Demux3/1 -> Fcn2/1  "x_H2O_in"
  x_in/1 -> Demux3/1
  Fcn/1 -> Sum1/1
  Fcn2/1 -> Sum1/2
  Fcn1/1 -> Sum2/1
  Fcn3/1 -> Sum2/2
  Sum2/1 -> Product6/2
  Sum1/1 -> Product5/2
  mdot_air/1 -> Product6/1, Product5/1  "mdot_air >=0"
  Product6/1 -> mdot_CO2/1
  Product5/1 -> mdot_H2O/1

== system carnotUIBK/HVAC/HVAC_2001_ventilation system simple/ventilation_zone 6/Subsystem ==
  note: (kg/s)
  note: (kg/s)
  note: (kg/s)
  note: (kg/kg)
  note: (kg/kg)
  note: ASSUMPTION: mdot_air_out2in = mdot_air_in2out !
  mdot_air : Inport
  x_in : Inport  Port=2
  x_out : Inport  Port=3
  Demux2 : Demux  Outputs=2
      settings: DisplayOption=none
  Demux3 : Demux  Outputs=2
      settings: DisplayOption=none
  Fcn{,1..3} (4 alike) : Fcn  Expr=u / (1+u)
  Product5 : Product  InputSameDT=on  SaturateOnIntegerOverflow=on  OutDataTypeStr=Inherit: Same as first input
  Product6 : Product  InputSameDT=on  SaturateOnIntegerOverflow=on  OutDataTypeStr=Inherit: Same as first input
  Sum1 : Sum  Inputs=+-  InputSameDT=on  SaturateOnIntegerOverflow=on  OutDataTypeStr=Inherit: Same as first input
  Sum2 : Sum  Inputs=+-  InputSameDT=on  SaturateOnIntegerOverflow=on  OutDataTypeStr=Inherit: Same as first input
  mdot_H2O : Outport  VectorParamsAs1DForOutWhenUnconnected=off
  mdot_CO2 : Outport  Port=2  VectorParamsAs1DForOutWhenUnconnected=off
  wires:
  x_out/1 -> Demux2/1
  Demux2/1 -> Fcn/1  "x_H2O_out"
  Demux2/2 -> Fcn1/1  "x_CO2_out"
  Demux3/2 -> Fcn3/1  "x_CO2_in"
  Demux3/1 -> Fcn2/1  "x_H2O_in"
  x_in/1 -> Demux3/1
  Fcn/1 -> Sum1/1
  Fcn2/1 -> Sum1/2
  Fcn1/1 -> Sum2/1
  Fcn3/1 -> Sum2/2
  Sum2/1 -> Product6/2
  Sum1/1 -> Product5/2
  mdot_air/1 -> Product6/1, Product5/1  "mdot_air >=0"
  Product6/1 -> mdot_CO2/1
  Product5/1 -> mdot_H2O/1

== system carnotUIBK/HVAC/HVAC_2001_ventilation system simple/ventilation_zone 7/Subsystem ==
  note: (kg/s)
  note: (kg/s)
  note: (kg/s)
  note: (kg/kg)
  note: (kg/kg)
  note: ASSUMPTION: mdot_air_out2in = mdot_air_in2out !
  mdot_air : Inport
  x_in : Inport  Port=2
  x_out : Inport  Port=3
  Demux2 : Demux  Outputs=2
      settings: DisplayOption=none
  Demux3 : Demux  Outputs=2
      settings: DisplayOption=none
  Fcn{,1..3} (4 alike) : Fcn  Expr=u / (1+u)
  Product5 : Product  InputSameDT=on  SaturateOnIntegerOverflow=on  OutDataTypeStr=Inherit: Same as first input
  Product6 : Product  InputSameDT=on  SaturateOnIntegerOverflow=on  OutDataTypeStr=Inherit: Same as first input
  Sum1 : Sum  Inputs=+-  InputSameDT=on  SaturateOnIntegerOverflow=on  OutDataTypeStr=Inherit: Same as first input
  Sum2 : Sum  Inputs=+-  InputSameDT=on  SaturateOnIntegerOverflow=on  OutDataTypeStr=Inherit: Same as first input
  mdot_H2O : Outport  VectorParamsAs1DForOutWhenUnconnected=off
  mdot_CO2 : Outport  Port=2  VectorParamsAs1DForOutWhenUnconnected=off
  wires:
  x_out/1 -> Demux2/1
  Demux2/1 -> Fcn/1  "x_H2O_out"
  Demux2/2 -> Fcn1/1  "x_CO2_out"
  Demux3/2 -> Fcn3/1  "x_CO2_in"
  Demux3/1 -> Fcn2/1  "x_H2O_in"
  x_in/1 -> Demux3/1
  Fcn/1 -> Sum1/1
  Fcn2/1 -> Sum1/2
  Fcn1/1 -> Sum2/1
  Fcn3/1 -> Sum2/2
  Sum2/1 -> Product6/2
  Sum1/1 -> Product5/2
  mdot_air/1 -> Product6/1, Product5/1  "mdot_air >=0"
  Product6/1 -> mdot_CO2/1
  Product5/1 -> mdot_H2O/1

== system carnotUIBK/HVAC/HVAC_2001_ventilation system simple/ventilation_zone 8/Subsystem ==
  note: (kg/s)
  note: (kg/s)
  note: (kg/s)
  note: (kg/kg)
  note: (kg/kg)
  note: ASSUMPTION: mdot_air_out2in = mdot_air_in2out !
  mdot_air : Inport
  x_in : Inport  Port=2
  x_out : Inport  Port=3
  Demux2 : Demux  Outputs=2
      settings: DisplayOption=none
  Demux3 : Demux  Outputs=2
      settings: DisplayOption=none
  Fcn{,1..3} (4 alike) : Fcn  Expr=u / (1+u)
  Product5 : Product  InputSameDT=on  SaturateOnIntegerOverflow=on  OutDataTypeStr=Inherit: Same as first input
  Product6 : Product  InputSameDT=on  SaturateOnIntegerOverflow=on  OutDataTypeStr=Inherit: Same as first input
  Sum1 : Sum  Inputs=+-  InputSameDT=on  SaturateOnIntegerOverflow=on  OutDataTypeStr=Inherit: Same as first input
  Sum2 : Sum  Inputs=+-  InputSameDT=on  SaturateOnIntegerOverflow=on  OutDataTypeStr=Inherit: Same as first input
  mdot_H2O : Outport  VectorParamsAs1DForOutWhenUnconnected=off
  mdot_CO2 : Outport  Port=2  VectorParamsAs1DForOutWhenUnconnected=off
  wires:
  x_out/1 -> Demux2/1
  Demux2/1 -> Fcn/1  "x_H2O_out"
  Demux2/2 -> Fcn1/1  "x_CO2_out"
  Demux3/2 -> Fcn3/1  "x_CO2_in"
  Demux3/1 -> Fcn2/1  "x_H2O_in"
  x_in/1 -> Demux3/1
  Fcn/1 -> Sum1/1
  Fcn2/1 -> Sum1/2
  Fcn1/1 -> Sum2/1
  Fcn3/1 -> Sum2/2
  Sum2/1 -> Product6/2
  Sum1/1 -> Product5/2
  mdot_air/1 -> Product6/1, Product5/1  "mdot_air >=0"
  Product6/1 -> mdot_CO2/1
  Product5/1 -> mdot_H2O/1

== system carnotUIBK/HVAC/HVAC_2001_ventilation system simple/ventilation_zone 9/Subsystem ==
  note: (kg/s)
  note: (kg/s)
  note: (kg/s)
  note: (kg/kg)
  note: (kg/kg)
  note: ASSUMPTION: mdot_air_out2in = mdot_air_in2out !
  mdot_air : Inport
  x_in : Inport  Port=2
  x_out : Inport  Port=3
  Demux2 : Demux  Outputs=2
      settings: DisplayOption=none
  Demux3 : Demux  Outputs=2
      settings: DisplayOption=none
  Fcn{,1..3} (4 alike) : Fcn  Expr=u / (1+u)
  Product5 : Product  InputSameDT=on  SaturateOnIntegerOverflow=on  OutDataTypeStr=Inherit: Same as first input
  Product6 : Product  InputSameDT=on  SaturateOnIntegerOverflow=on  OutDataTypeStr=Inherit: Same as first input
  Sum1 : Sum  Inputs=+-  InputSameDT=on  SaturateOnIntegerOverflow=on  OutDataTypeStr=Inherit: Same as first input
  Sum2 : Sum  Inputs=+-  InputSameDT=on  SaturateOnIntegerOverflow=on  OutDataTypeStr=Inherit: Same as first input
  mdot_H2O : Outport  VectorParamsAs1DForOutWhenUnconnected=off
  mdot_CO2 : Outport  Port=2  VectorParamsAs1DForOutWhenUnconnected=off
  wires:
  x_out/1 -> Demux2/1
  Demux2/1 -> Fcn/1  "x_H2O_out"
  Demux2/2 -> Fcn1/1  "x_CO2_out"
  Demux3/2 -> Fcn3/1  "x_CO2_in"
  Demux3/1 -> Fcn2/1  "x_H2O_in"
  x_in/1 -> Demux3/1
  Fcn/1 -> Sum1/1
  Fcn2/1 -> Sum1/2
  Fcn1/1 -> Sum2/1
  Fcn3/1 -> Sum2/2
  Sum2/1 -> Product6/2
  Sum1/1 -> Product5/2
  mdot_air/1 -> Product6/1, Product5/1  "mdot_air >=0"
  Product6/1 -> mdot_CO2/1
  Product5/1 -> mdot_H2O/1

== system carnotUIBK/HVAC/HVAC_9002_window opening/window opening 1/Transfer Fcn (with initial states) ==
  In1 : Inport
  State Space : StateSpace  A=A  B=B  C=C  D=Dd  InitialCondition=X0
  Out1 : Outport  InitialOutput=0  VectorParamsAs1DForOutWhenUnconnected=off
  wires:
  In1/1 -> State Space/1
  State Space/1 -> Out1/1

== system carnotUIBK/HVAC/HVAC_9002_window opening/window opening 1/Transfer Fcn (with initial states)1 ==
  In1 : Inport
  State Space : StateSpace  A=A  B=B  C=C  D=Dd  InitialCondition=X0
  Out1 : Outport  InitialOutput=0  VectorParamsAs1DForOutWhenUnconnected=off
  wires:
  State Space/1 -> Out1/1
  In1/1 -> State Space/1

== system carnotUIBK/HVAC/HVAC_9002_window opening/window opening 1/Transfer Fcn (with initial states)2 ==
  In1 : Inport
  State Space : StateSpace  A=A  B=B  C=C  D=Dd  InitialCondition=X0
  Out1 : Outport  InitialOutput=0  VectorParamsAs1DForOutWhenUnconnected=off
  wires:
  In1/1 -> State Space/1
  State Space/1 -> Out1/1

== system carnotUIBK/HVAC/HVAC_9002_window opening/window opening 2/Transfer Fcn (with initial states)1 ==
  In1 : Inport
  State Space : StateSpace  A=A  B=B  C=C  D=Dd  InitialCondition=X0
  Out1 : Outport  InitialOutput=0  VectorParamsAs1DForOutWhenUnconnected=off
  wires:
  State Space/1 -> Out1/1
  In1/1 -> State Space/1

== system carnotUIBK/HVAC/HVAC_9002_window opening/window opening 2/Transfer Fcn (with initial states)2 ==
  In1 : Inport
  State Space : StateSpace  A=A  B=B  C=C  D=Dd  InitialCondition=X0
  Out1 : Outport  InitialOutput=0  VectorParamsAs1DForOutWhenUnconnected=off
  wires:
  In1/1 -> State Space/1
  State Space/1 -> Out1/1

== system carnotUIBK/HVAC/HVAC_9002_window opening/window opening 2/Transfer Fcn (with initial states)3 ==
  In1 : Inport
  State Space : StateSpace  A=A  B=B  C=C  D=Dd  InitialCondition=X0
  Out1 : Outport  InitialOutput=0  VectorParamsAs1DForOutWhenUnconnected=off
  wires:
  In1/1 -> State Space/1
  State Space/1 -> Out1/1

== system carnotUIBK/HVAC/HVAC_9002_window opening/window opening 3/Transfer Fcn (with initial states)1 ==
  In1 : Inport
  State Space : StateSpace  A=A  B=B  C=C  D=Dd  InitialCondition=X0
  Out1 : Outport  InitialOutput=0  VectorParamsAs1DForOutWhenUnconnected=off
  wires:
  State Space/1 -> Out1/1
  In1/1 -> State Space/1

== system carnotUIBK/HVAC/HVAC_9002_window opening/window opening 3/Transfer Fcn (with initial states)2 ==
  In1 : Inport
  State Space : StateSpace  A=A  B=B  C=C  D=Dd  InitialCondition=X0
  Out1 : Outport  InitialOutput=0  VectorParamsAs1DForOutWhenUnconnected=off
  wires:
  In1/1 -> State Space/1
  State Space/1 -> Out1/1

== system carnotUIBK/HVAC/HVAC_9002_window opening/window opening 3/Transfer Fcn (with initial states)3 ==
  In1 : Inport
  State Space : StateSpace  A=A  B=B  C=C  D=Dd  InitialCondition=X0
  Out1 : Outport  InitialOutput=0  VectorParamsAs1DForOutWhenUnconnected=off
  wires:
  In1/1 -> State Space/1
  State Space/1 -> Out1/1

== system carnotUIBK/HVAC/HVAC_9002_window opening/window opening 4/Transfer Fcn (with initial states)1 ==
  In1 : Inport
  State Space : StateSpace  A=A  B=B  C=C  D=Dd  InitialCondition=X0
  Out1 : Outport  InitialOutput=0  VectorParamsAs1DForOutWhenUnconnected=off
  wires:
  State Space/1 -> Out1/1
  In1/1 -> State Space/1

== system carnotUIBK/HVAC/HVAC_9002_window opening/window opening 4/Transfer Fcn (with initial states)2 ==
  In1 : Inport
  State Space : StateSpace  A=A  B=B  C=C  D=Dd  InitialCondition=X0
  Out1 : Outport  InitialOutput=0  VectorParamsAs1DForOutWhenUnconnected=off
  wires:
  In1/1 -> State Space/1
  State Space/1 -> Out1/1

== system carnotUIBK/HVAC/HVAC_9002_window opening/window opening 4/Transfer Fcn (with initial states)3 ==
  In1 : Inport
  State Space : StateSpace  A=A  B=B  C=C  D=Dd  InitialCondition=X0
  Out1 : Outport  InitialOutput=0  VectorParamsAs1DForOutWhenUnconnected=off
  wires:
  In1/1 -> State Space/1
  State Space/1 -> Out1/1

== system carnotUIBK/HVAC/HVAC_9002_window opening/window opening 5/Transfer Fcn (with initial states)1 ==
  In1 : Inport
  State Space : StateSpace  A=A  B=B  C=C  D=Dd  InitialCondition=X0
  Out1 : Outport  InitialOutput=0  VectorParamsAs1DForOutWhenUnconnected=off
  wires:
  State Space/1 -> Out1/1
  In1/1 -> State Space/1

== system carnotUIBK/HVAC/HVAC_9002_window opening/window opening 5/Transfer Fcn (with initial states)2 ==
  In1 : Inport
  State Space : StateSpace  A=A  B=B  C=C  D=Dd  InitialCondition=X0
  Out1 : Outport  InitialOutput=0  VectorParamsAs1DForOutWhenUnconnected=off
  wires:
  In1/1 -> State Space/1
  State Space/1 -> Out1/1

== system carnotUIBK/HVAC/HVAC_9002_window opening/window opening 5/Transfer Fcn (with initial states)3 ==
  In1 : Inport
  State Space : StateSpace  A=A  B=B  C=C  D=Dd  InitialCondition=X0
  Out1 : Outport  InitialOutput=0  VectorParamsAs1DForOutWhenUnconnected=off
  wires:
  In1/1 -> State Space/1
  State Space/1 -> Out1/1

== system carnotUIBK/HVAC/HVAC_9002_window opening/window opening 6/Transfer Fcn (with initial states)1 ==
  In1 : Inport
  State Space : StateSpace  A=A  B=B  C=C  D=Dd  InitialCondition=X0
  Out1 : Outport  InitialOutput=0  VectorParamsAs1DForOutWhenUnconnected=off
  wires:
  State Space/1 -> Out1/1
  In1/1 -> State Space/1

== system carnotUIBK/HVAC/HVAC_9002_window opening/window opening 6/Transfer Fcn (with initial states)2 ==
  In1 : Inport
  State Space : StateSpace  A=A  B=B  C=C  D=Dd  InitialCondition=X0
  Out1 : Outport  InitialOutput=0  VectorParamsAs1DForOutWhenUnconnected=off
  wires:
  In1/1 -> State Space/1
  State Space/1 -> Out1/1

== system carnotUIBK/HVAC/HVAC_9002_window opening/window opening 6/Transfer Fcn (with initial states)3 ==
  In1 : Inport
  State Space : StateSpace  A=A  B=B  C=C  D=Dd  InitialCondition=X0
  Out1 : Outport  InitialOutput=0  VectorParamsAs1DForOutWhenUnconnected=off
  wires:
  In1/1 -> State Space/1
  State Space/1 -> Out1/1

== system carnotUIBK/gain/People/W//ppl (activity)/LUT_Qdot_dry ==
  note: SENSITIVE/DRY HEAT POWER emitted from a person in a room
  activity : Inport
  Top : Inport  Port=2
  Look-Up Table Qdot_dry : Subsystem  mask(Lookup Table (2-D)){x=[10 12 14 16 18 20 22 23 24 25 26 28 30 32 34], y=[0 1 2 3 4], t=[135 135 135 170 210; 125 125 125 160 195; 115 115 115 150 180; 105 105 105 135 165; 100 100 100 125 152; 95 95 95 115 140; 90 90 90 105 125; 85 85 85 100 117; 80 80 80 95 110; 75 75 75 90 102; 70 70 70 85 95; 60 60 60 70 80; 50 50 50 60 65; 30 30 30 35 40; 0 0 0 0 0]}
      mask prompts: x "Row:"; y "Column:"; t "Table:"
      mask help: Performs 2-D linear interpolation of input values using the specified input/output table. Extrapolation is performed outside the table boundaries.
      mask init:
      | [r,c]=size(t);
      | x=reshape(x,prod(size(x)),1);
      | xi=x(:,ones(1,c));
      | minx=min(x); maxx=max(x);
      | mint=min(min(t)); maxt=max(max(t));
      mask Display: plot(xi,t,[minx maxx],[mint mint],[minx minx],[mint maxt])
  Qdot_dry : Outport  InitialOutput=0  VectorParamsAs1DForOutWhenUnconnected=off
  wires:
  activity/1 -> Look-Up Table Qdot_dry/2(Cols)
  Look-Up Table Qdot_dry/1(U) -> Qdot_dry/1
  Top/1 -> Look-Up Table Qdot_dry/1(Rows)
